simulink model "lead_and_resistance"  (Simulink 7.4)
settings: Solver=ode45  StartTime=0.0  StopTime=1e-2  MaxStep=1e-7
settings Model: Creator=Administrator  LastModifiedBy=Administrator

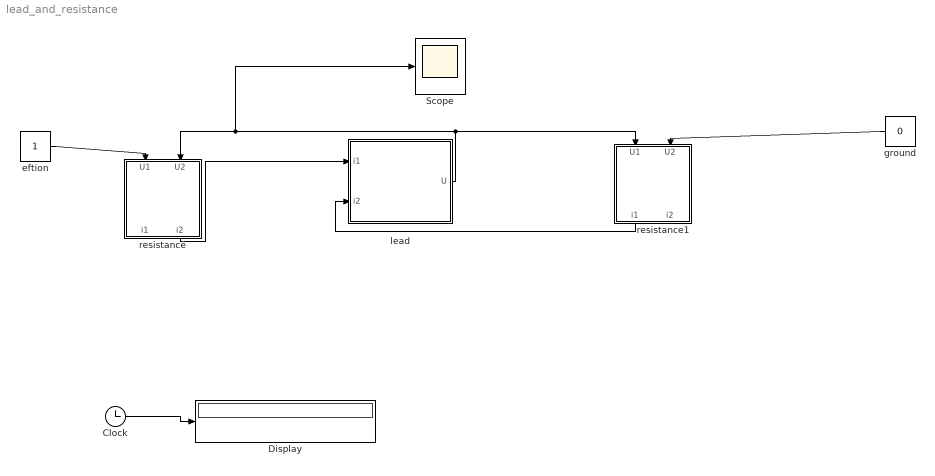
== system lead_and_resistance ==
  Clock : Clock
      settings: Decimation=10
  Display : Display
  Scope : Scope
      settings: YMin=-11000  YMax=-1000
  eftion : Constant  OutDataType=fixdt(1, 16)  OutScaling=2^0
  ground : Constant  Value=0  OutDataType=fixdt(1, 16)  OutScaling=2^0
  lead : Subsystem
  resistance : Subsystem
  resistance1 : Subsystem
  wires:
  resistance/2(i2) -> lead/1(i1)
  resistance1/1(i1) -> lead/2(i2)
  ground/1 -> resistance1/2(U2)
  lead/1(U) -> resistance1/1(U1), resistance/2(U2), Scope/1
  eftion/1 -> resistance/1(U1)
  Clock/1 -> Display/1

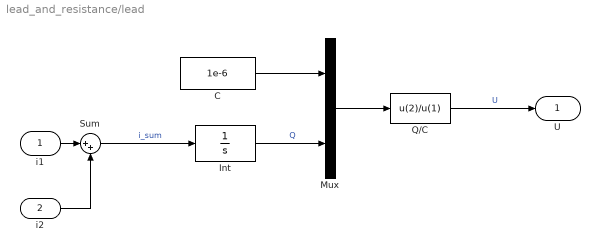
== system lead_and_resistance/lead ==
  i1 : Inport
  i2 : Inport  Port=2
  C : Constant  Value=1e-6  OutDataType=fixdt(1, 16)  OutScaling=2^0
  Int : Integrator
  Mux : Mux  Inputs=2
  Q/C : Fcn  Expr=u(2)/u(1)
  Sum : Sum  Inputs=|++  OutDataType=fixdt(1, 16)  OutScaling=2^0
  U : Outport
  wires:
  Sum/1 -> Int/1  "i_sum"
  Mux/1 -> Q/C/1
  C/1 -> Mux/1
  Int/1 -> Mux/2  "Q"
  Q/C/1 -> U/1  "U"
  i1/1 -> Sum/1
  i2/1 -> Sum/2

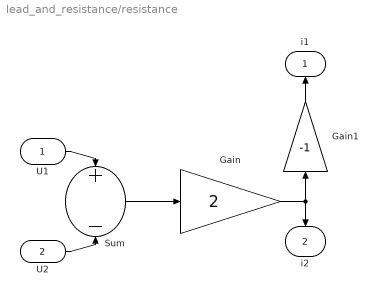
== system lead_and_resistance/resistance ==
  U1 : Inport
  U2 : Inport  Port=2
  Gain : Gain  Gain=2  ParameterDataType=fixdt(1, 16)  ParameterScaling=2^0  OutDataType=fixdt(1, 16)  OutScaling=2^0
  Gain1 : Gain  Gain=-1  ParameterDataType=fixdt(1, 16)  ParameterScaling=2^0  OutDataType=fixdt(1, 16)  OutScaling=2^0
  Sum : Sum  Inputs=+|-  OutDataType=fixdt(1, 16)  OutScaling=2^0
  i1 : Outport
  i2 : Outport  Port=2
  wires:
  Sum/1 -> Gain/1
  Gain/1 -> Gain1/1, i2/1
  Gain1/1 -> i1/1
  U1/1 -> Sum/1
  U2/1 -> Sum/2

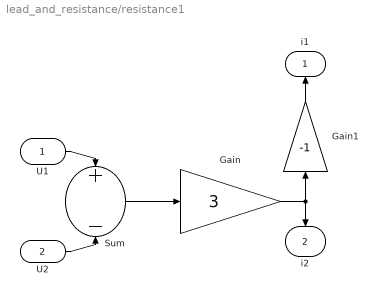
== system lead_and_resistance/resistance1 ==
  U1 : Inport
  U2 : Inport  Port=2
  Gain : Gain  Gain=3  ParameterDataType=fixdt(1, 16)  ParameterScaling=2^0  OutDataType=fixdt(1, 16)  OutScaling=2^0
  Gain1 : Gain  Gain=-1  ParameterDataType=fixdt(1, 16)  ParameterScaling=2^0  OutDataType=fixdt(1, 16)  OutScaling=2^0
  Sum : Sum  Inputs=+|-  OutDataType=fixdt(1, 16)  OutScaling=2^0
  i1 : Outport
  i2 : Outport  Port=2
  wires:
  Sum/1 -> Gain/1
  Gain/1 -> Gain1/1, i2/1
  Gain1/1 -> i1/1
  U1/1 -> Sum/1
  U2/1 -> Sum/2
